simulink model "DSQPID_test"  (Simulink 5.0)
settings: Solver=ode45  StartTime=0.0  StopTime=2  FixedStep=0.001  RelTol=1e-3
settings Model: LastModifiedBy=ThinkPad  RTWOptions="-aEnforceIntegerDowncast=1 -aExtMode=0 -aExtModeTesting=0 -aFoldNonRolledExpr=1 -aForceParamTrailComments=0 -aGenerateComments=1 -aGenerateReport=0 -aIgnoreCustomStorageClasses=1 -aIncDataTypeInIds=0 -aIncHierarchyInIds=0 -aInlineInvariantSignals=0 -aInlinedPrmAccess=\"Literals\" -aLocalBlockOutputs=1 -aLogVarNameModifier=\"rt_\" -aMaxRTWIdLen=31 -aPrefixModelToSubsysFcnNames=1 -aRTWVerbose=1 -aRollThreshold=5 -aShowEliminatedStatements=0"

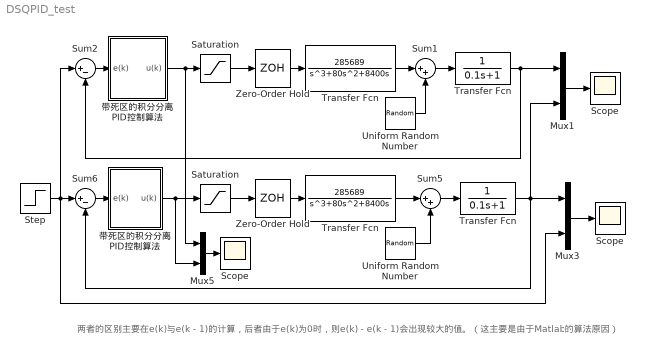
== system DSQPID_test ==
  note: 两者的区别主要在e(k)与e(k－1)的计算，后者由于e(k)为0时，则e(k)－e(k－1)会出现较大的值。（这主要是由于Matlab的算法原因）
  " Scope " : Scope
      settings: YMin=-2  YMax=10  SaveName=DSQPIDtestu  DataFormat=Array  MaxDataPoints=500000
  " Transfer Fcn" : TransferFcn  Denominator=[0.1 1]
  " Transfer Fcn " : TransferFcn  Denominator=[0.1 1]
  Mux1 : Mux  Inputs=2
  Mux3 : Mux  Inputs=2
  Mux5 : Mux  Inputs=2
  Saturation : Saturate  UpperLimit=10  LowerLimit=-10
  "Saturation " : Saturate  UpperLimit=10  LowerLimit=-10
  Scope : Scope
      settings: YMin=0.955  YMax=1.035  SaveName=DSQPIDy  DataFormat=Array  MaxDataPoints=500000
  "Scope " : Scope
      settings: YMin=0.955  YMax=1.035  SaveName=DSQPIDtesty  DataFormat=Array  MaxDataPoints=500000
  Step : Step  Time=0  SampleTime=0
  Sum1 : Sum  Inputs=|++  SaturateOnIntegerOverflow=on
  Sum2 : Sum  Inputs=|+-  SaturateOnIntegerOverflow=on
  Sum5 : Sum  Inputs=|++  SaturateOnIntegerOverflow=on
  Sum6 : Sum  Inputs=|+-  SaturateOnIntegerOverflow=on
  Transfer Fcn : TransferFcn  Numerator=[285689]  Denominator=[1 80 8400 0]
  "Transfer Fcn " : TransferFcn  Numerator=[285689]  Denominator=[1 80 8400 0]
  Uniform Random Number : UniformRandomNumber  Minimum=-0.5  Maximum=0.5  SampleTime=0
  "Uniform Random Number " : UniformRandomNumber  Minimum=-0.5  Maximum=0.5  SampleTime=0
  Zero-Order Hold : ZeroOrderHold  SampleTime=0.001
  "Zero-Order Hold " : ZeroOrderHold  SampleTime=0.001
  带死区的积分分离 PID控制算法 : Subsystem
  "带死区的积分分离 PID控制算法  " : Subsystem
  wires:
  "Transfer Fcn "/1 -> Sum5/1
  Sum5/1 -> " Transfer Fcn"/1
  Uniform Random Number/1 -> Sum5/2
  带死区的积分分离 PID控制算法/1(u(k)) -> "Saturation "/1, Mux5/2
  Mux3/1 -> Scope/1
  " Transfer Fcn"/1 -> Mux3/1, Sum6/2, Mux1/2
  "Zero-Order Hold "/1 -> "Transfer Fcn "/1
  Mux5/1 -> " Scope "/1
  Step/1 -> Mux3/2, Sum2/1, Sum6/1
  "Saturation "/1 -> "Zero-Order Hold "/1
  Transfer Fcn/1 -> Sum1/1
  Sum1/1 -> " Transfer Fcn "/1
  "Uniform Random Number "/1 -> Sum1/2
  "带死区的积分分离 PID控制算法  "/1(u(k)) -> Saturation/1, Mux5/1
  Mux1/1 -> "Scope "/1
  " Transfer Fcn "/1 -> Sum2/2, Mux1/1
  Zero-Order Hold/1 -> Transfer Fcn/1
  Saturation/1 -> Zero-Order Hold/1
  Sum2/1 -> "带死区的积分分离 PID控制算法  "/1(e(k))
  Sum6/1 -> 带死区的积分分离 PID控制算法/1(e(k))

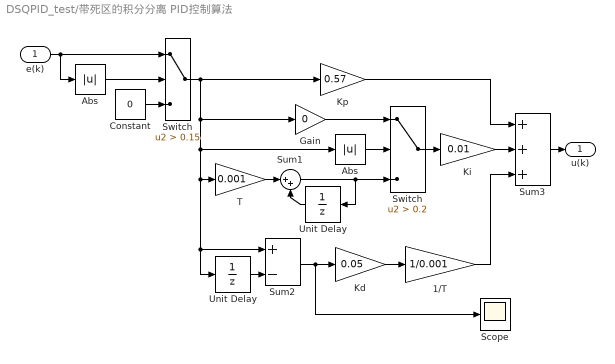
== system DSQPID_test/带死区的积分分离 PID控制算法 ==
  e(k) : Inport
  1/T : Gain  Gain=1/0.001  SaturateOnIntegerOverflow=on
  Abs : Abs  SaturateOnIntegerOverflow=on
  "Abs " : Abs  SaturateOnIntegerOverflow=on
  "Constant " : Constant  Value=0
  Gain : Gain  Gain=0  SaturateOnIntegerOverflow=on
  Kd : Gain  Gain=0.05  SaturateOnIntegerOverflow=on
  Ki : Gain  Gain=0.01  SaturateOnIntegerOverflow=on
  Kp : Gain  Gain=0.57  SaturateOnIntegerOverflow=on
  "Scope " : Scope
      settings: YMin=-2  YMax=10  SaveName=DSQPIDu1  DataFormat=Array  MaxDataPoints=500000
  Sum1 : Sum  Inputs=|++  SaturateOnIntegerOverflow=on
  Sum2 : Sum  Inputs=+-  SaturateOnIntegerOverflow=on
  Sum3 : Sum  Inputs=+++  SaturateOnIntegerOverflow=on
  Switch : Switch  Criteria=u2 > Threshold  Threshold=0.2  SaturateOnIntegerOverflow=on  InputSameDT=on
  "Switch " : Switch  Criteria=u2 > Threshold  Threshold=0.15  SaturateOnIntegerOverflow=on  InputSameDT=on
  T : Gain  Gain=0.001  SaturateOnIntegerOverflow=on
  Unit Delay : UnitDelay  SampleTime=0.001
  "Unit Delay " : UnitDelay  Orientation=left  SampleTime=0.001
  u(k) : Outport
  wires:
  Ki/1 -> Sum3/2
  Switch/1 -> Ki/1
  1/T/1 -> Sum3/3
  Kd/1 -> 1/T/1
  Kp/1 -> Sum3/1
  e(k)/1 -> "Switch "/1, "Abs "/1
  Sum2/1 -> Kd/1, "Scope "/1
  Gain/1 -> Switch/1
  Abs/1 -> Switch/2
  T/1 -> Sum1/1
  "Unit Delay "/1 -> Sum1/2
  Sum1/1 -> "Unit Delay "/1, Switch/3
  Sum3/1 -> u(k)/1
  "Abs "/1 -> "Switch "/2
  "Constant "/1 -> "Switch "/3
  "Switch "/1 -> Kp/1, Gain/1, Abs/1, T/1, Sum2/1, Unit Delay/1
  Unit Delay/1 -> Sum2/2

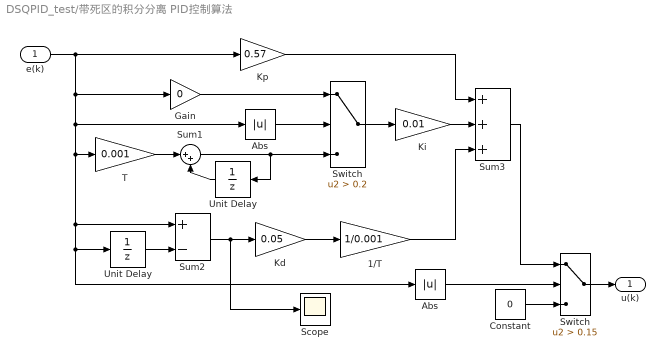
== system DSQPID_test/带死区的积分分离 PID控制算法   ==
  e(k) : Inport
  1/T : Gain  Gain=1/0.001  SaturateOnIntegerOverflow=on
  Abs : Abs  SaturateOnIntegerOverflow=on
  "Abs " : Abs  SaturateOnIntegerOverflow=on
  "Constant " : Constant  Value=0
  Gain : Gain  Gain=0  SaturateOnIntegerOverflow=on
  Kd : Gain  Gain=0.05  SaturateOnIntegerOverflow=on
  Ki : Gain  Gain=0.01  SaturateOnIntegerOverflow=on
  Kp : Gain  Gain=0.57  SaturateOnIntegerOverflow=on
  Scope : Scope
      settings: YMin=-2  YMax=10  SaveName=DSQPIDu2  DataFormat=Array  MaxDataPoints=500000
  Sum1 : Sum  Inputs=|++  SaturateOnIntegerOverflow=on
  Sum2 : Sum  Inputs=+-  SaturateOnIntegerOverflow=on
  Sum3 : Sum  Inputs=+++  SaturateOnIntegerOverflow=on
  Switch : Switch  Criteria=u2 > Threshold  Threshold=0.2  SaturateOnIntegerOverflow=on  InputSameDT=on
  "Switch " : Switch  Criteria=u2 > Threshold  Threshold=0.15  SaturateOnIntegerOverflow=on  InputSameDT=on
  T : Gain  Gain=0.001  SaturateOnIntegerOverflow=on
  Unit Delay : UnitDelay  SampleTime=0.001
  "Unit Delay " : UnitDelay  Orientation=left  SampleTime=0.001
  u(k) : Outport
  wires:
  "Switch "/1 -> u(k)/1
  "Constant "/1 -> "Switch "/3
  "Abs "/1 -> "Switch "/2
  Sum1/1 -> Switch/3, "Unit Delay "/1
  "Unit Delay "/1 -> Sum1/2
  T/1 -> Sum1/1
  Abs/1 -> Switch/2
  Gain/1 -> Switch/1
  Sum2/1 -> Kd/1, Scope/1
  e(k)/1 -> Gain/1, Sum2/1, "Abs "/1, Unit Delay/1, T/1, Abs/1, Kp/1
  Kp/1 -> Sum3/1
  Kd/1 -> 1/T/1
  1/T/1 -> Sum3/3
  Switch/1 -> Ki/1
  Ki/1 -> Sum3/2
  Sum3/1 -> "Switch "/1
  Unit Delay/1 -> Sum2/2
